simulink model "ex4sima"  (R2015a)
settings: Solver=ode45  StartTime=0.0  StopTime=tf  RelTol=1e-3
values from neighbouring files (symbols this model uses):
  A = [0, 1; 0, 0]    [ex4.m]
  B = [0; -m*g*d/(L*(J/R^2 + m))]    [ex4.m]
  C = K*(s+a)/s    [ex1.m]    (also in ex4.m = [1, 0])
settings Model: Creator=BPeixoto  LastModifiedBy=BPeixoto

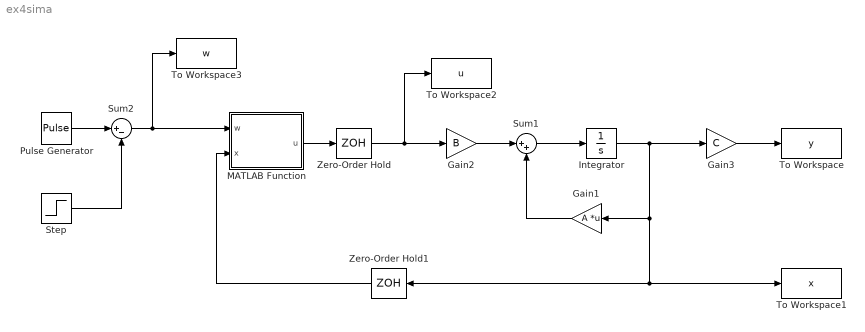
== system ex4sima ==
  Gain1 : Gain  Gain=A  Multiplication=Matrix(K*u)
  Gain2 : Gain  Gain=B
  Gain3 : Gain  Gain=C
  Integrator : Integrator
  MATLAB Function : MATLAB Function  TreatAsAtomicUnit=on
  Pulse Generator : DiscretePulseGenerator  PulseType=Time based  Amplitude=0.2  Period=20  PulseWidth=50
  Step : Step  Time=0  After=0.2  SampleTime=0
  Sum1 : Sum  Inputs=|++
  Sum2 : Sum  Inputs=|+-
  To Workspace : ToWorkspace  VariableName=y  SaveFormat=Structure With Time  SampleTime=-1
  To Workspace1 : ToWorkspace  VariableName=x  SaveFormat=Structure With Time  SampleTime=-1
  To Workspace2 : ToWorkspace  VariableName=u  SaveFormat=Structure With Time  SampleTime=-1
  To Workspace3 : ToWorkspace  VariableName=w  SaveFormat=Structure With Time  SampleTime=-1
  Zero-Order Hold : ZeroOrderHold
  Zero-Order Hold1 : ZeroOrderHold
  wires:
  Sum1/1 -> Integrator/1
  Gain2/1 -> Sum1/1
  Gain3/1 -> To Workspace/1
  Gain1/1 -> Sum1/2
  Pulse Generator/1 -> Sum2/1
  Step/1 -> Sum2/2
  Sum2/1 -> To Workspace3/1, MATLAB Function/1(w)
  Integrator/1 -> Gain3/1, To Workspace1/1, Zero-Order Hold1/1, Gain1/1
  MATLAB Function/1(u) -> Zero-Order Hold/1
  Zero-Order Hold/1 -> To Workspace2/1, Gain2/1
  Zero-Order Hold1/1 -> MATLAB Function/2(x)

== matlab function ex4sima/MATLAB Function ==
  data: u output; w input; x input; params parameter
function u = fcn(w, x, params)   
    u = -params.K*x + params.F*w;
